simulink model "DPF_Regeneration"  (Simulink 9.1)
settings: Solver=FixedStepDiscrete  StartTime=0.0  StopTime=60  FixedStep=1  RelTol=1e-3
settings Model: Creator=Kore  LastModifiedBy=Kore
settings DataIOCC: SaveFormat=Dataset  ReturnWorkspaceOutputs=on
settings OptimizationCC: LifeSpan=auto
settings DebuggingCC: UnderspecifiedInitializationDetection=Simplified  MergeDetectMultiDrivingBlocksExec=error  SFUnexpectedBacktrackingDiag=error  SFNoUnconditionalDefaultTransitionDiag=error  SFExecutionAtInitializationDiag=warning
settings HardwareCC: ProdBitPerPointer=64  ProdBitPerSizeT=64  ProdBitPerPtrDiffT=64  ProdLargestAtomicFloat=Float  ProdIntDivRoundTo=Zero  ProdEndianess=LittleEndian  ProdWordSize=64  ProdHWDeviceType=Intel->x86-64 (Windows64)
settings ModelReferenceCC: PropagateSignalLabelsOutOfModel=on
settings SFSimCC: SimUseLocalCustomCode=on
settings RTWCC: RTWUseLocalCustomCode=on
settings CodeAppCC: StateflowObjectComments=off
settings GRTTargetCC: TargetLangStandard=C99 (ISO)  CombineOutputUpdateFcns=on  GRTInterface=off
settings ConfigComp: CovMetricSettings=dwe  CovHtmlReporting=off  CovSaveCumulativeToWorkspaceVar=off  CovSaveSingleToWorkspaceVar=off  CovExternalEMLEnable=on

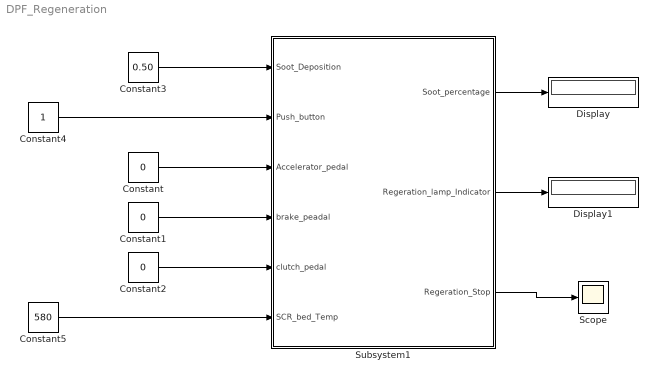
== system DPF_Regeneration ==
  Constant : Constant  Value=0
  Constant1 : Constant  Value=0
  Constant2 : Constant  Value=0
  Constant3 : Constant  Value=0.50
  Constant4 : Constant
  Constant5 : Constant  Value=580
  Display : Display
  Display1 : Display
  Scope : Scope
  Subsystem1 : Subsystem
  wires:
  Constant1/1 -> Subsystem1/4("brake_peadal ")
  Constant/1 -> Subsystem1/3(Accelerator_pedal)
  Constant2/1 -> Subsystem1/5(clutch_pedal)
  Constant3/1 -> Subsystem1/1(Soot_Deposition)
  Subsystem1/3(Regeration_Stop) -> Scope/1
  Constant4/1 -> Subsystem1/2(Push_button)
  Constant5/1 -> Subsystem1/6(SCR_bed_Temp)
  Subsystem1/1(Soot_percentage) -> Display/1
  Subsystem1/2(Regeration_lamp_Indicator) -> Display1/1

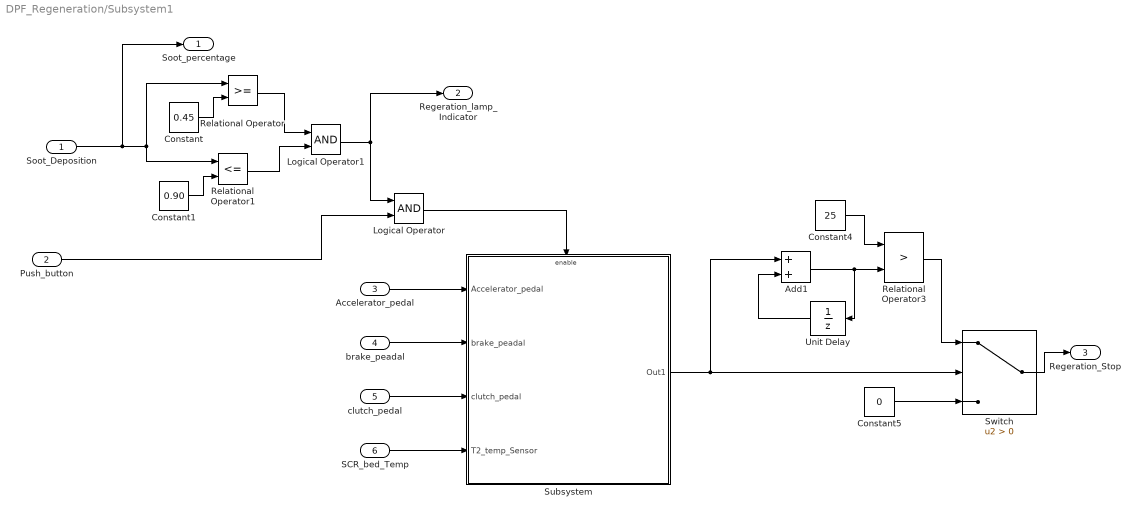
== system DPF_Regeneration/Subsystem1 ==
  Soot_Deposition : Inport
  Push_button : Inport  Port=2
  Accelerator_pedal : Inport  Port=3
  "brake_peadal " : Inport  Port=4
  clutch_pedal : Inport  Port=5
  SCR_bed_Temp : Inport  Port=6
  Add1 : Sum
  Constant : Constant  Value=0.45
  Constant1 : Constant  Value=0.90
  Constant4 : Constant  Value=25
  Constant5 : Constant  Value=0
  Logical Operator : Logic  AllPortsSameDT=off  OutDataTypeStr=boolean
  Logical Operator1 : Logic  AllPortsSameDT=off  OutDataTypeStr=boolean
  Relational Operator : RelationalOperator  OutDataTypeStr=boolean  RndMeth=Simplest
  Relational Operator1 : RelationalOperator  Operator=<=  OutDataTypeStr=boolean  RndMeth=Simplest
  Relational Operator3 : RelationalOperator  Operator=>  OutDataTypeStr=boolean  RndMeth=Simplest
  Subsystem : Subsystem
  Switch : Switch  Criteria=u2 > Threshold
  Unit Delay : UnitDelay  SampleTime=-1  HasFrameUpgradeWarning=on
  Soot_percentage : Outport
  Regeration_lamp_Indicator : Outport  Port=2
  Regeration_Stop : Outport  Port=3
  wires:
  Soot_Deposition/1 -> Soot_percentage/1, Relational Operator1/1, Relational Operator/1
  clutch_pedal/1 -> Subsystem/3(clutch_pedal)
  Logical Operator1/1 -> Regeration_lamp_Indicator/1, Logical Operator/1
  Push_button/1 -> Logical Operator/2
  SCR_bed_Temp/1 -> Subsystem/4(T2_temp_Sensor)
  "brake_peadal "/1 -> Subsystem/2("brake_peadal ")
  Constant/1 -> Relational Operator/2
  Subsystem/1(Out1) -> Add1/1, Switch/2
  Constant1/1 -> Relational Operator1/2
  Accelerator_pedal/1 -> Subsystem/1(Accelerator_pedal)
  Logical Operator/1 -> Subsystem/Enable
  Unit Delay/1 -> Add1/2
  Add1/1 -> Unit Delay/1, Relational Operator3/2
  Constant4/1 -> Relational Operator3/1
  Constant5/1 -> Switch/3
  Switch/1 -> Regeration_Stop/1
  Relational Operator3/1 -> Switch/1
  Relational Operator/1 -> Logical Operator1/1
  Relational Operator1/1 -> Logical Operator1/2

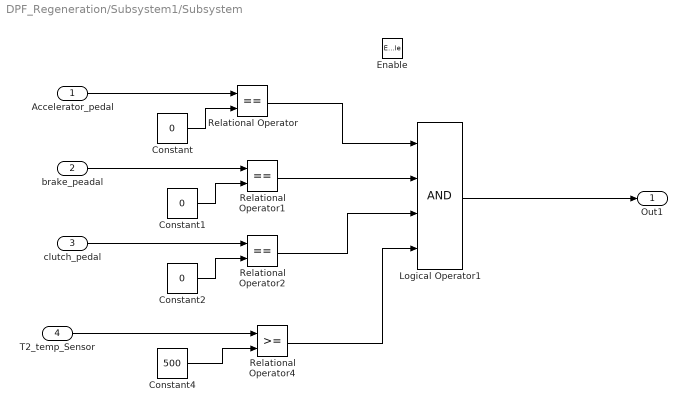
== system DPF_Regeneration/Subsystem1/Subsystem ==
  Accelerator_pedal : Inport
  "brake_peadal " : Inport  Port=2
  clutch_pedal : Inport  Port=3
  T2_temp_Sensor : Inport  Port=4
  Enable : EnablePort  StatesWhenEnabling=reset
  Constant : Constant  Value=0
  Constant1 : Constant  Value=0
  Constant2 : Constant  Value=0
  Constant4 : Constant  Value=500
  Logical Operator1 : Logic  Inputs=4  AllPortsSameDT=off  OutDataTypeStr=boolean
  Relational Operator : RelationalOperator  Operator===  OutDataTypeStr=boolean  RndMeth=Simplest
  Relational Operator1 : RelationalOperator  Operator===  OutDataTypeStr=boolean  RndMeth=Simplest
  Relational Operator2 : RelationalOperator  Operator===  OutDataTypeStr=boolean  RndMeth=Simplest
  Relational Operator4 : RelationalOperator  OutDataTypeStr=boolean  RndMeth=Simplest
  Out1 : Outport
  wires:
  Constant/1 -> Relational Operator/2
  Accelerator_pedal/1 -> Relational Operator/1
  "brake_peadal "/1 -> Relational Operator1/1
  Constant1/1 -> Relational Operator1/2
  Constant2/1 -> Relational Operator2/2
  clutch_pedal/1 -> Relational Operator2/1
  Relational Operator/1 -> Logical Operator1/1
  Relational Operator1/1 -> Logical Operator1/2
  Relational Operator2/1 -> Logical Operator1/3
  T2_temp_Sensor/1 -> Relational Operator4/1
  Constant4/1 -> Relational Operator4/2
  Logical Operator1/1 -> Out1/1
  Relational Operator4/1 -> Logical Operator1/4
